simulink model "RightArmAgent"  (Simulink 6.5)
settings: Solver=ode45  SolverMode=SingleTasking  StartTime=0.0  StopTime=10.0  RelTol=1e-3  AbsTol=1e-6
settings Model: Creator=The MathWorks Inc.  LastModifiedBy=suarezjl  ExtModeTrigMode=oneshot  ExtModeArmWhenConnect=off  ExtModeAutoUpdateStatusClock=off
settings DataIOCC: LimitDataPoints=off  SignalLoggingName=logsOut
settings OptimizationCC: BooleanDataType=off  InlineInvariantSignals=on
settings DebuggingCC: CheckExecutionContextPreStartOutputMsg=on  CheckExecutionContextRuntimeOutputMsg=on  SolverPrmCheckMsg=none  MultiTaskDSMMsg=warning  MultiTaskCondExecSysMsg=none  IntegerOverflowMsg=none  StrictBusMsg=None
settings HardwareCC: TargetUnknown=on
settings ModelReferenceCC: UpdateModelReferenceTargets=IfOutOfDate
settings RTWCC: IncludeERTFirstTime=on

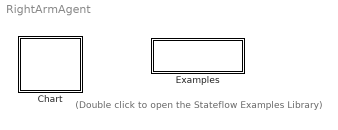
== system RightArmAgent ==
  note: (Double click to open the
      | Stateflow Examples Library)
  Chart : Stateflow chart
  Examples : Subsystem
      settings: OpenFcn=sf('Private','sf_examples')
      mask Display: disp('Examples')

== system RightArmAgent/Examples ==

== stateflow chart Chart ==
  state InitialArmRoutine
    Popeye\RightArm\HomingController.ComputeHomingPressures()
    Popeye\RightArm\SampleIndPressure.HW_IO_6()
    Popeye\RightArm\StateMachine.Wait(50)
  state InitializeFunctions
    Popeye\RightArm\HomingController.Initial()
    Popeye\RightArm\SampleIndPressure.Initialize()
    Popeye\RightArm\PIDNonLinCtrl.Initial()
    Popeye\RightArm\ForwardKinematics.Initialize()
    Popeye\RightArm\InverseKinematics.Initialize()
    Popeye\RightArm\SampleIndPressure.Disable_ZMasking()
  state WriteHomeDesiredLogicalAngles
    Popeye\RightArm\SampleIndPressure.Enable_ZMasking()
    Popeye\RightArm\SampleIndPressure.WriteHomePositions()
  state LoadHomePosition
    Popeye\RightArm\SampleIndPressure.HW_IO_6()
    Popeye\RightArm\PIDNonLinCtrl.PID_NonLin_6Press()
    Popeye\RightArm\ForwardKinematics.ForwardKinematics()
    Popeye\RightArm\InverseKinematics.InverseKinematics()
  state PID_NonLinCtrlLoop
    Popeye\RightArm\Filter.FilterDesiredAngles()
    Popeye\RightArm\PIDNonLinCtrl.PID_NonLin_12Press()
    Popeye\RightArm\SampleIndPressure.HW_IO_12()
    Popeye\RightArm\PIDNonLinCtrl.Read_CurrentPressure()
    Popeye\RightArm\ForwardKinematics.ForwardKinematics()
    Popeye\RightArm\InverseKinematics.InverseKinematics()
    Popeye\RightArm\StateMachine.Wait(50)
  state Stop
    Popeye\RightArm\SampleIndPressure.Reset()
  (default) -> InitializeFunctions : Start
  InitialArmRoutine -> InitialArmRoutine [order 1] : Default
  InitializeFunctions -> InitialArmRoutine : Always
  WriteHomeDesiredLogicalAngles -> LoadHomePosition : Always
  LoadHomePosition -> PID_NonLinCtrlLoop : Always
  InitialArmRoutine -> WriteHomeDesiredLogicalAngles [order 2] : Signal="Go to next state"
  PID_NonLinCtrlLoop -> PID_NonLinCtrlLoop [order 1] : Default
  PID_NonLinCtrlLoop -> Stop [order 2] : Signal="Stop"
